simulink model "sysgen_oversample2x_2samples_per_clock"  (R2016b)
settings: Solver=VariableStepAuto  StartTime=0.0  StopTime=samples_per_channel*number_channels/Fadc  RelTol=1e-3
PreLoadFcn:
  | setup
values from neighbouring files (symbols this model uses):
  Fadc = 614e6    (= 614000000)    [setup.m]
undefined symbols (not defined in the file or in its folder): j
libraries: xbsIndex_r4 x434, dspsigops x2, hdlsllib x2
(part 1 of 4)
settings Model: Creator=mdewart  LastModifiedBy=mdewart

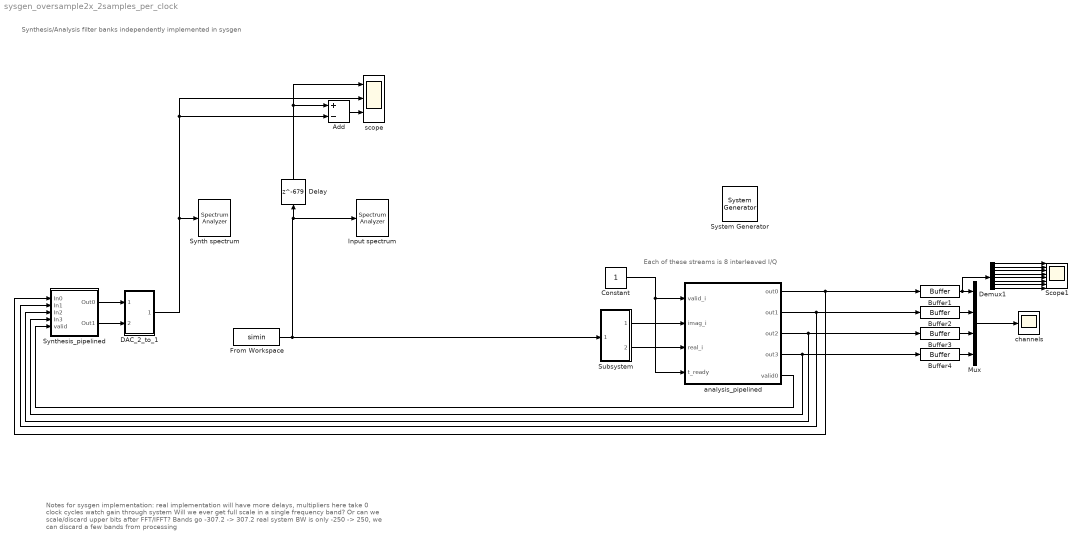
== system sysgen_oversample2x_2samples_per_clock ==
  note: Synthesis/Analysis filter banks independently implemented in sysgen
  note: Notes for sysgen implementation:
      |
      | real implementation will have more delays, multipliers here take 0 clock cycles
      |
      | watch gain through system
      |      Will we ever get full scale in a single frequency band?  Or can we scale/discard upper bits after FFT/IFFT?
      |
      | Bands go -307.2 -> 307.2  real system BW is only -250 -> 250, we can discard a few bands from processing
  note: Each of these streams is 8 interleaved I/Q
  " System Generator" : xbsIndex_r4/ System Generator  Tag=genX  xilinxfamily=kintexu  part=xcku040  speed=-2-e  package=ffva1156  synthesis_tool=Vivado  clock_wrapper=Clock Enables  directory=./netlist  proj_type=Vivado  Synth_file=Vivado Synthesis Defaults  Impl_file=Vivado Implementation Defaults  testbench=off  simulink_period=2/Fadc  sysclk_period=2e9/Fadc  dcm_input_clock_period=10  incr_netlist=off  trim_vbits=Everywhere in SubSystem  dbl_ovrd=According to Block Masks  core_generation=According to Block Masks  run_coregen=off  deprecated_control=off  eval_field=0  block_type=sysgen
  Add : Sum  Inputs=+-
  Buffer{1..4} (4 alike) : Buffer  N=8  TreatMby1Signals=One channel  OutputFrames=off
  Constant : Constant  SampleTime=2/Fadc
  DAC_2_to_1 : Subsystem
  Delay : Delay  DelayLength=679  InitialCondition=0
  Demux1 : Demux  Outputs=8
  From Workspace : FromWorkspace  VariableName=simin  SampleTime=1/Fadc  Interpolate=off  OutputAfterFinalValue=Cyclic repetition
  Input spectrum : SpectrumAnalyzer
  Mux : Mux
  Scope1 : Scope  NumInputPorts=8
  Subsystem : Subsystem
  Synth spectrum : SpectrumAnalyzer
  Synthesis_pipelined : Subsystem  VariantControl=Variant
  analysis_pipelined : Subsystem
  channels : Scope
  scope : Scope  NumInputPorts=3
  wires:
  Mux/1 -> channels/1
  Buffer2/1 -> Mux/2
  Buffer3/1 -> Mux/3
  Buffer4/1 -> Mux/4
  DAC_2_to_1/1(Out1) -> scope/2, Add/2, Synth spectrum/1
  Delay/1 -> Add/1, scope/1
  Subsystem/1(imag) -> analysis_pipelined/2(imag_i)
  Subsystem/2(real) -> analysis_pipelined/3(real_i)
  Constant/1 -> analysis_pipelined/4(t_ready), analysis_pipelined/1(valid_i)
  Buffer1/1 -> Demux1/1, Mux/1
  From Workspace/1 -> Input spectrum/1, Delay/1, Subsystem/1(In1)
  Demux1/1 -> Scope1/1
  Demux1/2 -> Scope1/2
  Demux1/3 -> Scope1/3
  Demux1/4 -> Scope1/4
  Demux1/5 -> Scope1/5
  Demux1/6 -> Scope1/6
  Demux1/7 -> Scope1/7
  Demux1/8 -> Scope1/8
  analysis_pipelined/3(out2) -> Synthesis_pipelined/3(In2), Buffer3/1
  analysis_pipelined/4(out3) -> Synthesis_pipelined/4(In3), Buffer4/1
  analysis_pipelined/2(out1) -> Synthesis_pipelined/2(In1), Buffer2/1
  analysis_pipelined/1(out0) -> Synthesis_pipelined/1(In0), Buffer1/1
  Synthesis_pipelined/1(Out0) -> DAC_2_to_1/1(In1)
  Synthesis_pipelined/2(Out1) -> DAC_2_to_1/2(In2)
  analysis_pipelined/5(valid0) -> Synthesis_pipelined/5(valid)
  Add/1 -> scope/3

== system sysgen_oversample2x_2samples_per_clock/DAC_2_to_1 ==
  In1 : Inport
  In2 : Inport  Port=2
  Add2 : Sum
  Delay7 : Delay  DelayLength=1  InitialCondition=0
  Gain : Gain  Gain=16
  Upsample1 : dspsigops/Upsample  N=2  phase=0  RateOptions=Allow multirate processing  ic=0  mode=Unused parameter value
  Upsample2 : dspsigops/Upsample  N=2  phase=0  RateOptions=Allow multirate processing  ic=0  mode=Unused parameter value
  Out1 : Outport
  wires:
  In2/1 -> Upsample2/1
  Delay7/1 -> Add2/2
  In1/1 -> Upsample1/1
  Upsample1/1 -> Add2/1
  Add2/1 -> Gain/1
  Upsample2/1 -> Delay7/1
  Gain/1 -> Out1/1

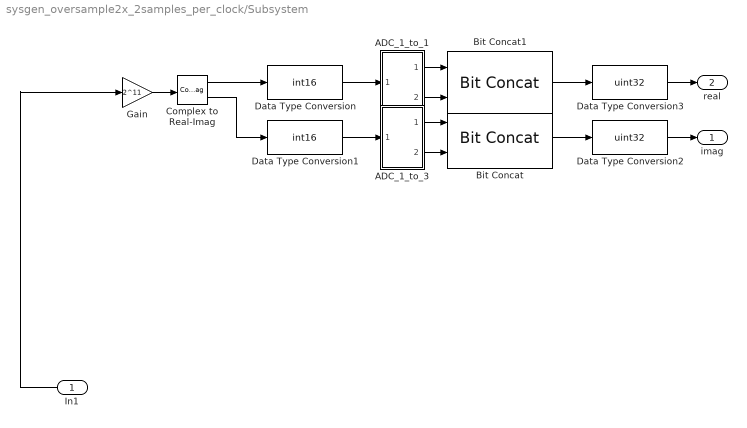
== system sysgen_oversample2x_2samples_per_clock/Subsystem ==
  In1 : Inport
  ADC_1_to_1 : Subsystem
  ADC_1_to_3 : Subsystem
  Bit Concat : hdlsllib/HDL Operations/Bit Concat  numInputs=2
  Bit Concat1 : hdlsllib/HDL Operations/Bit Concat  numInputs=2
  Complex to Real-Imag : ComplexToRealImag
  Data Type Conversion : DataTypeConversion  OutDataTypeStr=int16
  Data Type Conversion1 : DataTypeConversion  OutDataTypeStr=int16
  Data Type Conversion2 : DataTypeConversion  OutDataTypeStr=uint32  ConvertRealWorld=Stored Integer (SI)
  Data Type Conversion3 : DataTypeConversion  OutDataTypeStr=uint32  ConvertRealWorld=Stored Integer (SI)
  Gain : Gain  Gain=2^11
  imag : Outport
  real : Outport  Port=2
  wires:
  In1/1 -> Gain/1
  Data Type Conversion/1 -> ADC_1_to_1/1(In1)
  Complex to Real-Imag/1 -> Data Type Conversion/1
  ADC_1_to_3/2(Out2) -> Bit Concat/2
  Data Type Conversion1/1 -> ADC_1_to_3/1(In1)
  ADC_1_to_1/1(Out1) -> Bit Concat1/1
  Bit Concat/1 -> Data Type Conversion2/1
  ADC_1_to_3/1(Out1) -> Bit Concat/1
  ADC_1_to_1/2(Out2) -> Bit Concat1/2
  Complex to Real-Imag/2 -> Data Type Conversion1/1
  Gain/1 -> Complex to Real-Imag/1
  Bit Concat1/1 -> Data Type Conversion3/1
  Data Type Conversion2/1 -> imag/1
  Data Type Conversion3/1 -> real/1

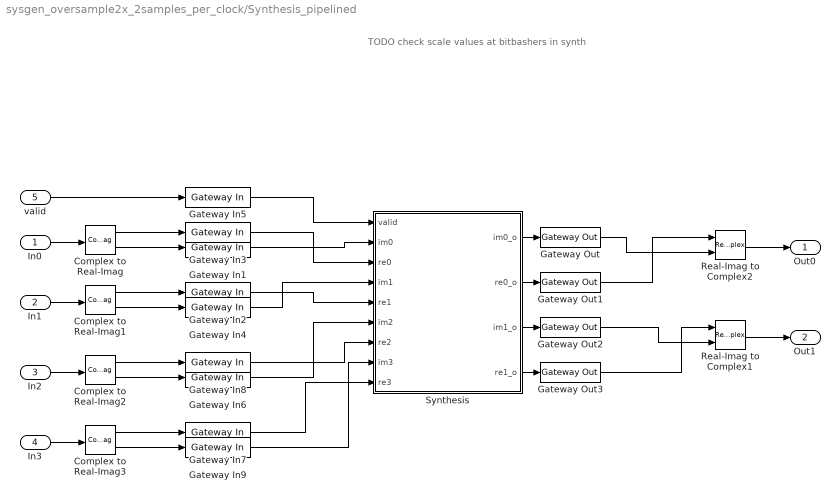
== system sysgen_oversample2x_2samples_per_clock/Synthesis_pipelined ==
  note: TODO check scale values at bitbashers in synth
  In0 : Inport
  In1 : Inport  Port=2
  In2 : Inport  Port=3
  In3 : Inport  Port=4
  valid : Inport  Port=5
  Complex to Real-Imag{,1..3} (4 alike) : ComplexToRealImag
  Gateway In{1..4,6..9} (8 alike) : xbsIndex_r4/Gateway In  gui_display_data_type=Fixed-point  arith_type="Signed  (2's comp)"  n_bits=16  bin_pt=15  preci_type=Single  exp_width=8  frac_width=24  rows=1  columns=1  quantization="Round  (unbiased: +/- Inf)"  overflow=Saturate  period=2/Fadc  UseAsADC=off  ADCChannel='1'  interface=None  automatic_assignment=on  address_offset=hex2dec('00')  intf_name=''  intf_description=''  default_value=0  timing_constraint=None  locs_specified=off  LOCs={}  io_standard={}  inherit_from_input=off  hdl_port=on  dbl_ovrd=off  block_type=gatewayin
  Gateway In5 : xbsIndex_r4/Gateway In  gui_display_data_type=Boolean  arith_type=Boolean  n_bits=1  bin_pt=0  preci_type=Single  exp_width=8  frac_width=24  rows=1  columns=1  quantization="Round  (unbiased: +/- Inf)"  overflow=Saturate  period=2/Fadc  UseAsADC=off  ADCChannel='1'  interface=None  automatic_assignment=on  address_offset=hex2dec('00')  intf_name=''  intf_description=''  default_value=0  timing_constraint=None  locs_specified=off  LOCs={}  io_standard={}  inherit_from_input=off  hdl_port=on  dbl_ovrd=off  block_type=gatewayin
  Gateway Out{,1..3} (4 alike) : xbsIndex_r4/Gateway Out  inherit_from_input=off  hdl_port=on  rows=1  columns=1  UseAsDAC=off  DACChannel='1'  interface=None  automatic_assignment=on  address_offset=hex2dec('00')  intf_name=''  intf_description=''  timing_constraint=None  locs_specified=off  LOCs={}  io_standard={}  block_type=gatewayout
  Real-Imag to Complex1 : RealImagToComplex
  Real-Imag to Complex2 : RealImagToComplex
  Synthesis : Subsystem
  Out0 : Outport
  Out1 : Outport  Port=2
  wires:
  Real-Imag to Complex1/1 -> Out1/1
  Real-Imag to Complex2/1 -> Out0/1
  Gateway Out3/1 -> Real-Imag to Complex1/1
  Gateway Out2/1 -> Real-Imag to Complex1/2
  Gateway Out/1 -> Real-Imag to Complex2/2
  Gateway Out1/1 -> Real-Imag to Complex2/1
  Synthesis/4(re1_o) -> Gateway Out3/1
  Synthesis/3(im1_o) -> Gateway Out2/1
  Synthesis/2(re0_o) -> Gateway Out1/1
  Synthesis/1(im0_o) -> Gateway Out/1
  Gateway In7/1 -> Synthesis/9(re3)
  Gateway In9/1 -> Synthesis/8(im3)
  Gateway In8/1 -> Synthesis/7(re2)
  Gateway In6/1 -> Synthesis/6(im2)
  Gateway In4/1 -> Synthesis/4(im1)
  Gateway In2/1 -> Synthesis/5(re1)
  Gateway In5/1 -> Synthesis/1(valid)
  Gateway In1/1 -> Synthesis/2(im0)
  Gateway In3/1 -> Synthesis/3(re0)
  In2/1 -> Complex to Real-Imag2/1
  In3/1 -> Complex to Real-Imag3/1
  Complex to Real-Imag3/2 -> Gateway In9/1
  Complex to Real-Imag3/1 -> Gateway In7/1
  Complex to Real-Imag2/2 -> Gateway In6/1
  Complex to Real-Imag2/1 -> Gateway In8/1
  In0/1 -> Complex to Real-Imag/1
  In1/1 -> Complex to Real-Imag1/1
  Complex to Real-Imag1/2 -> Gateway In4/1
  Complex to Real-Imag1/1 -> Gateway In2/1
  Complex to Real-Imag/2 -> Gateway In1/1
  Complex to Real-Imag/1 -> Gateway In3/1
  valid/1 -> Gateway In5/1

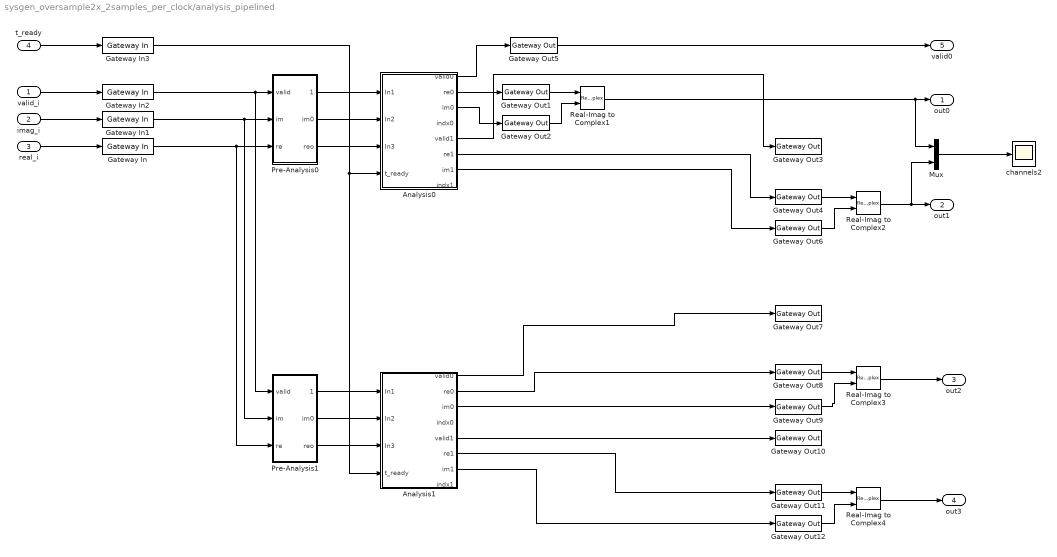
== system sysgen_oversample2x_2samples_per_clock/analysis_pipelined ==
  valid_i : Inport
  imag_i : Inport  Port=2
  real_i : Inport  Port=3
  t_ready : Inport  Port=4
  Analysis0 : Subsystem
  Analysis1 : Subsystem
  Gateway In : xbsIndex_r4/Gateway In  gui_display_data_type=Fixed-point  arith_type=Unsigned  n_bits=32  bin_pt=0  preci_type=Single  exp_width=8  frac_width=24  rows=1  columns=1  quantization="Round  (unbiased: +/- Inf)"  overflow=Saturate  period=2/Fadc  UseAsADC=off  ADCChannel='1'  interface=None  automatic_assignment=on  address_offset=hex2dec('00')  intf_name=''  intf_description=''  default_value=0  timing_constraint=None  locs_specified=off  LOCs={}  io_standard={}  inherit_from_input=off  hdl_port=on  dbl_ovrd=off  block_type=gatewayin
  Gateway In1 : xbsIndex_r4/Gateway In  gui_display_data_type=Fixed-point  arith_type=Unsigned  n_bits=32  bin_pt=0  preci_type=Single  exp_width=8  frac_width=24  rows=1  columns=1  quantization="Round  (unbiased: +/- Inf)"  overflow=Saturate  period=2/Fadc  UseAsADC=off  ADCChannel='1'  interface=None  automatic_assignment=on  address_offset=hex2dec('00')  intf_name=''  intf_description=''  default_value=0  timing_constraint=None  locs_specified=off  LOCs={}  io_standard={}  inherit_from_input=off  hdl_port=on  dbl_ovrd=off  block_type=gatewayin
  Gateway In2 : xbsIndex_r4/Gateway In  gui_display_data_type=Boolean  arith_type=Boolean  n_bits=1  bin_pt=0  preci_type=Single  exp_width=8  frac_width=24  rows=1  columns=1  quantization="Round  (unbiased: +/- Inf)"  overflow=Saturate  period=2/Fadc  UseAsADC=off  ADCChannel='1'  interface=None  automatic_assignment=on  address_offset=hex2dec('00')  intf_name=''  intf_description=''  default_value=0  timing_constraint=None  locs_specified=off  LOCs={}  io_standard={}  inherit_from_input=off  hdl_port=on  dbl_ovrd=off  block_type=gatewayin
  Gateway In3 : xbsIndex_r4/Gateway In  gui_display_data_type=Boolean  arith_type=Boolean  n_bits=1  bin_pt=0  preci_type=Single  exp_width=8  frac_width=24  rows=1  columns=1  quantization="Round  (unbiased: +/- Inf)"  overflow=Saturate  period=2/Fadc  UseAsADC=off  ADCChannel='1'  interface=None  automatic_assignment=on  address_offset=hex2dec('00')  intf_name=''  intf_description=''  default_value=0  timing_constraint=None  locs_specified=off  LOCs={}  io_standard={}  inherit_from_input=off  hdl_port=on  dbl_ovrd=off  block_type=gatewayin
  Gateway Out{1..12} (12 alike) : xbsIndex_r4/Gateway Out  inherit_from_input=off  hdl_port=on  rows=1  columns=1  UseAsDAC=off  DACChannel='1'  interface=None  automatic_assignment=on  address_offset=hex2dec('00')  intf_name=''  intf_description=''  timing_constraint=None  locs_specified=off  LOCs={}  io_standard={}  block_type=gatewayout
  Mux : Mux  Inputs=2
  Pre-Analysis0 : Subsystem
  Pre-Analysis1 : Subsystem
  Real-Imag to Complex{1..4} (4 alike) : RealImagToComplex
  channels2 : Scope
  out0 : Outport
  out1 : Outport  Port=2
  out2 : Outport  Port=3
  out3 : Outport  Port=4
  valid0 : Outport  Port=5
  wires:
  Gateway In2/1 -> Pre-Analysis0/1(valid), Pre-Analysis1/1(valid)
  Analysis1/7(im1) -> Gateway Out12/1
  Analysis1/6(re1) -> Gateway Out11/1
  Analysis1/3(im0) -> Gateway Out9/1
  Analysis0/1(valid0) -> Gateway Out5/1
  Analysis0/2(re0) -> Gateway Out1/1
  Analysis0/3(im0) -> Gateway Out2/1
  Real-Imag to Complex4/1 -> out3/1
  Real-Imag to Complex3/1 -> out2/1
  Real-Imag to Complex1/1 -> Mux/1, out0/1
  Gateway Out5/1 -> valid0/1
  Pre-Analysis1/1(valid0) -> Analysis1/1(In1)
  Pre-Analysis1/2(im0) -> Analysis1/2(In2)
  Pre-Analysis1/3(reo) -> Analysis1/3(In3)
  Gateway In3/1 -> Analysis0/4(t_ready), Analysis1/4(t_ready)
  Pre-Analysis0/1(valid0) -> Analysis0/1(In1)
  Pre-Analysis0/2(im0) -> Analysis0/2(In2)
  Pre-Analysis0/3(reo) -> Analysis0/3(In3)
  Gateway In/1 -> Pre-Analysis0/3(re), Pre-Analysis1/3(re)
  Gateway In1/1 -> Pre-Analysis0/2(im), Pre-Analysis1/2(im)
  Analysis1/5(valid1) -> Gateway Out10/1
  Analysis1/2(re0) -> Gateway Out8/1
  Analysis1/1(valid0) -> Gateway Out7/1
  Gateway Out9/1 -> Real-Imag to Complex3/2
  Gateway Out8/1 -> Real-Imag to Complex3/1
  Gateway Out12/1 -> Real-Imag to Complex4/2
  Gateway Out11/1 -> Real-Imag to Complex4/1
  Analysis0/7(im1) -> Gateway Out6/1
  Analysis0/6(re1) -> Gateway Out4/1
  Analysis0/5(valid1) -> Gateway Out3/1
  Gateway Out2/1 -> Real-Imag to Complex1/2
  Gateway Out1/1 -> Real-Imag to Complex1/1
  Gateway Out6/1 -> Real-Imag to Complex2/2
  Gateway Out4/1 -> Real-Imag to Complex2/1
  imag_i/1 -> Gateway In1/1
  real_i/1 -> Gateway In/1
  t_ready/1 -> Gateway In3/1
  valid_i/1 -> Gateway In2/1
  Real-Imag to Complex2/1 -> Mux/2, out1/1
  Mux/1 -> channels2/1

== system sysgen_oversample2x_2samples_per_clock/Subsystem/ADC_1_to_1 ==
  In1 : Inport
  Delay1 : Delay  DelayLength=1  InitialCondition=0
  Downsample : DownSample  RateOptions=Allow multirate processing
  Downsample1 : DownSample  RateOptions=Allow multirate processing
  Out1 : Outport
  Out2 : Outport  Port=2
  wires:
  Downsample/1 -> Out2/1
  In1/1 -> Downsample/1, Delay1/1
  Downsample1/1 -> Out1/1
  Delay1/1 -> Downsample1/1

== system sysgen_oversample2x_2samples_per_clock/Subsystem/ADC_1_to_3 ==
  In1 : Inport
  Delay1 : Delay  DelayLength=1  InitialCondition=0
  Downsample : DownSample  RateOptions=Allow multirate processing
  Downsample1 : DownSample  RateOptions=Allow multirate processing
  Out1 : Outport
  Out2 : Outport  Port=2
  wires:
  Delay1/1 -> Downsample1/1
  Downsample1/1 -> Out1/1
  In1/1 -> Delay1/1, Downsample/1
  Downsample/1 -> Out2/1

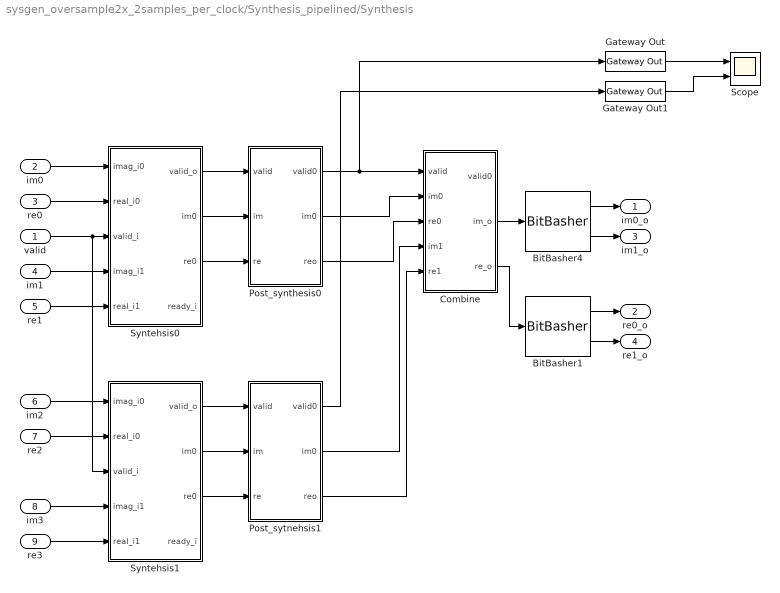
== system sysgen_oversample2x_2samples_per_clock/Synthesis_pipelined/Synthesis ==
  valid : Inport
  im0 : Inport  Port=2
  re0 : Inport  Port=3
  im1 : Inport  Port=4
  re1 : Inport  Port=5
  im2 : Inport  Port=6
  re2 : Inport  Port=7
  im3 : Inport  Port=8
  re3 : Inport  Port=9
  BitBasher1 : xbsIndex_r4/BitBasher  bitexpr=|  display_expr=off  sr_1=hi  arith_type1="Signed  (2's comp)"  bin_pt1=15  sr_2=lo  arith_type2="Signed  (2's comp)"  bin_pt2=15  sr_3=hi  arith_type3=Unsigned  bin_pt3=0  sr_4=4  arith_type4=Unsigned  bin_pt4=0  dbl_ovrd=off  block_type=bitbasher
      | hi = {in[31:16]}
      | lo = {in[15:0]}
  BitBasher4 : xbsIndex_r4/BitBasher  bitexpr=|  display_expr=off  sr_1=hi  arith_type1="Signed  (2's comp)"  bin_pt1=15  sr_2=lo  arith_type2="Signed  (2's comp)"  bin_pt2=15  sr_3=hi  arith_type3=Unsigned  bin_pt3=0  sr_4=4  arith_type4=Unsigned  bin_pt4=0  dbl_ovrd=off  block_type=bitbasher
      | hi = {in[31:16]}
      | lo = {in[15:0]}
  Combine : Subsystem
  Gateway Out : xbsIndex_r4/Gateway Out  inherit_from_input=off  hdl_port=off  rows=1  columns=1  UseAsDAC=off  DACChannel='1'  interface=None  automatic_assignment=on  address_offset=hex2dec('00')  intf_name=''  intf_description=''  timing_constraint=None  locs_specified=off  LOCs={}  io_standard={}  block_type=gatewayout
  Gateway Out1 : xbsIndex_r4/Gateway Out  inherit_from_input=off  hdl_port=off  rows=1  columns=1  UseAsDAC=off  DACChannel='1'  interface=None  automatic_assignment=on  address_offset=hex2dec('00')  intf_name=''  intf_description=''  timing_constraint=None  locs_specified=off  LOCs={}  io_standard={}  block_type=gatewayout
  Post_synthesis0 : Subsystem
  Post_sytnehsis1 : Subsystem
  Scope : Scope  NumInputPorts=2
  Syntehsis0 : Subsystem
  Syntehsis1 : Subsystem
  im0_o : Outport
  re0_o : Outport  Port=2
  im1_o : Outport  Port=3
  re1_o : Outport  Port=4
  wires:
  Post_sytnehsis1/1(valid0) -> Gateway Out1/1
  Gateway Out1/1 -> Scope/2
  Gateway Out/1 -> Scope/1
  Syntehsis0/1(valid_o) -> Post_synthesis0/1(valid)
  BitBasher1/2 -> re1_o/1
  BitBasher1/1 -> re0_o/1
  BitBasher4/2 -> im1_o/1
  BitBasher4/1 -> im0_o/1
  Combine/3(re_o) -> BitBasher1/1
  Combine/2(im_o) -> BitBasher4/1
  Post_sytnehsis1/3(reo) -> Combine/5(re1)
  Post_sytnehsis1/2(im0) -> Combine/4(im1)
  Post_synthesis0/3(reo) -> Combine/3(re0)
  Post_synthesis0/2(im0) -> Combine/2(im0)
  Post_synthesis0/1(valid0) -> Combine/1(valid), Gateway Out/1
  Syntehsis0/3(re0) -> Post_synthesis0/3(re)
  Syntehsis0/2(im0) -> Post_synthesis0/2(im)
  Syntehsis1/1(valid_o) -> Post_sytnehsis1/1(valid)
  Syntehsis1/3(re0) -> Post_sytnehsis1/3(re)
  Syntehsis1/2(im0) -> Post_sytnehsis1/2(im)
  im3/1 -> Syntehsis1/4(imag_i1)
  re1/1 -> Syntehsis0/5(real_i1)
  valid/1 -> Syntehsis1/3(valid_i), Syntehsis0/3(valid_i)
  re3/1 -> Syntehsis1/5(real_i1)
  im1/1 -> Syntehsis0/4(imag_i1)
  im0/1 -> Syntehsis0/1(imag_i0)
  re0/1 -> Syntehsis0/2(real_i0)
  re2/1 -> Syntehsis1/2(real_i0)
  im2/1 -> Syntehsis1/1(imag_i0)

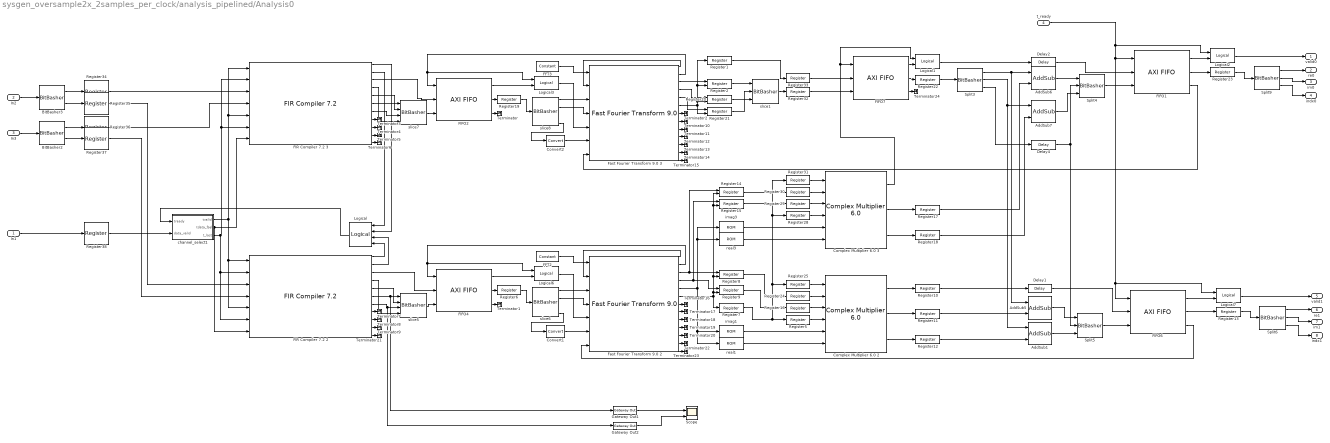
== system sysgen_oversample2x_2samples_per_clock/analysis_pipelined/Analysis0 ==
  In1 : Inport
  In2 : Inport  Port=2
  In3 : Inport  Port=3
  t_ready : Inport  Port=4
  AddSub{1,5..7} (4 alike) : xbsIndex_r4/AddSub  mode=Addition  use_carryin=off  use_carryout=off  en=off  latency=2  precision=Full  arith_type="Signed  (2's comp)"  n_bits=22  bin_pt=16  quantization=Truncate  overflow=Wrap  use_behavioral_HDL=on  hw_selection=Fabric  pipelined=off  dbl_ovrd=off  block_type=addsub
  BitBasher2 : xbsIndex_r4/BitBasher  bitexpr=|  display_expr=off  sr_1=hi  arith_type1="Signed  (2's comp)"  bin_pt1=15  sr_2=lo  arith_type2="Signed  (2's comp)"  bin_pt2=15  sr_3=hi  arith_type3=Unsigned  bin_pt3=0  sr_4=4  arith_type4=Unsigned  bin_pt4=0  dbl_ovrd=off  block_type=bitbasher
      | hi = {in[31:16]}
      | lo = {in[15:0]}
  BitBasher3 : xbsIndex_r4/BitBasher  bitexpr=|  display_expr=off  sr_1=hi  arith_type1="Signed  (2's comp)"  bin_pt1=15  sr_2=lo  arith_type2="Signed  (2's comp)"  bin_pt2=15  sr_3=hi  arith_type3=Unsigned  bin_pt3=0  sr_4=4  arith_type4=Unsigned  bin_pt4=0  dbl_ovrd=off  block_type=bitbasher
      | hi = {in[31:16]}
      | lo = {in[15:0]}
  Complex Multiplier 6.0 2 : xbsIndex_r4/Complex Multiplier 6.0   hasatlast=off  hasatuser=off  atuserwidth=1  hasbtlast=off  hasbtuser=off  btuserwidth=1  multtype=Use_Mults  optimizegoal=Performance  flowcontrol=NonBlocking  outputwidth=24  roundmode=Truncate  hasctrltlast=off  hasctrltuser=off  ctrltuserwidth=1  outtlastbehv=Null  latencyconfig=Automatic  minimumlatency=34  aclken=off  aresetn=off  trim_axipin_name=on  simulation_type=hybrid_sim  simulation_model=sysgen:cmpy_v6_0  data_path_portlist={ 's_axis_a_tdata_real', 's_axis_a_tdata_imag', 's_axis_b_tdata_real', 's_axis_b_tdata_imag', 's_axis_ctrl_tdata_rounding_bit', 'm_axis_dout_tdata_real', 'm_axis_dout_tdata_imag' }  aportwidth=63  bportwidth=63  ip_name=Complex Multiplier  ip_version=6.0  dsptool_ready=true  ipcore_usecache=true  ipcore_useipmodelcache=true  ipcore_verbose=false  ipcore_latency_parameter='minimumlatency'  wrapper_available=true  port_translation_map={ 'aclken' => 'en', 'aresetn' => 'rst'}  block_type=cmpy_v6_0
  Complex Multiplier 6.0 3 : xbsIndex_r4/Complex Multiplier 6.0   hasatlast=off  hasatuser=off  atuserwidth=1  hasbtlast=off  hasbtuser=off  btuserwidth=1  multtype=Use_Mults  optimizegoal=Performance  flowcontrol=NonBlocking  outputwidth=24  roundmode=Truncate  hasctrltlast=off  hasctrltuser=off  ctrltuserwidth=1  outtlastbehv=Null  latencyconfig=Automatic  minimumlatency=34  aclken=off  aresetn=off  trim_axipin_name=on  simulation_type=hybrid_sim  simulation_model=sysgen:cmpy_v6_0  data_path_portlist={ 's_axis_a_tdata_real', 's_axis_a_tdata_imag', 's_axis_b_tdata_real', 's_axis_b_tdata_imag', 's_axis_ctrl_tdata_rounding_bit', 'm_axis_dout_tdata_real', 'm_axis_dout_tdata_imag' }  aportwidth=63  bportwidth=63  ip_name=Complex Multiplier  ip_version=6.0  dsptool_ready=true  ipcore_usecache=true  ipcore_useipmodelcache=true  ipcore_verbose=false  ipcore_latency_parameter='minimumlatency'  wrapper_available=true  port_translation_map={ 'aclken' => 'en', 'aresetn' => 'rst'}  block_type=cmpy_v6_0
  Convert1 : xbsIndex_r4/Convert  gui_display_data_type=Boolean  arith_type=Boolean  n_bits=16  bin_pt=15  float_type=Single  exp_bits=8  fraction_bits=24  quantization=Truncate  overflow=Flag as error  en=off  latency=0  pipeline=off  dbl_ovrd=off  block_type=convert
  Convert2 : xbsIndex_r4/Convert  gui_display_data_type=Boolean  arith_type=Boolean  n_bits=16  bin_pt=15  float_type=Single  exp_bits=8  fraction_bits=24  quantization=Truncate  overflow=Flag as error  en=off  latency=0  pipeline=off  dbl_ovrd=off  block_type=convert
  Delay1 : xbsIndex_r4/Delay  rst=off  infoeditControl=Selection of Reset will increase slice count due to use of real FFs and instead of SRLs  en=off  latency=2  reg_retiming=on  dbl_ovrd=off  block_type=delay
  Delay2 : xbsIndex_r4/Delay  rst=off  infoeditControl=Selection of Reset will increase slice count due to use of real FFs and instead of SRLs  en=off  latency=2  reg_retiming=on  dbl_ovrd=off  block_type=delay
  Delay4 : xbsIndex_r4/Delay  rst=off  infoeditControl=Selection of Reset will increase slice count due to use of real FFs and instead of SRLs  en=off  latency=2  reg_retiming=on  dbl_ovrd=off  block_type=delay
  FFT2 : xbsIndex_r4/Constant  const=1  gui_display_data_type=Fixed-point  arith_type=Unsigned  n_bits=1  bin_pt=0  preci_type=Single  exp_width=8  frac_width=24  explicit_period=off  period=1  equ=P=C  opselect=C  inp2=PCIN>>17  opr=+  inp1=P  carry=CIN  dbl_ovrd=off  block_type=constant
  FFT3 : xbsIndex_r4/Constant  const=1  gui_display_data_type=Fixed-point  arith_type=Unsigned  n_bits=1  bin_pt=0  preci_type=Single  exp_width=8  frac_width=24  explicit_period=off  period=1  equ=P=C  opselect=C  inp2=PCIN>>17  opr=+  inp1=P  carry=CIN  dbl_ovrd=off  block_type=constant
  FIFO{1..2,4,6} (4 alike) : xbsIndex_r4/AXI FIFO  input_depth_axis=16  actual_fifo_depth_label=18  enable_tdata=on  enable_tdest=off  enable_tstrb=off  enable_tready=on  enable_tid=off  enable_tuser=off  enable_tkeep=off  enable_tlast=off  has_aresetn=off  enable_data_counts_axis=off  fifo_implementation_type_axis=Common Clock Distributed RAM  trim_axipin_name=on  programmable_full_type_axis=Full  full_threshold_assert_value_axis=0  programmable_empty_type_axis=Empty  empty_threshold_assert_value_axis=1022  underflow_flag_axi=0  underflow_sense_axi=Active High  overflow_flag_axi=0  overflow_sense_axi=Active High  block_type=axi_fifo
  FIFO7 : xbsIndex_r4/AXI FIFO  input_depth_axis=32  actual_fifo_depth_label=34  enable_tdata=on  enable_tdest=off  enable_tstrb=off  enable_tready=on  enable_tid=off  enable_tuser=off  enable_tkeep=off  enable_tlast=off  has_aresetn=off  enable_data_counts_axis=off  fifo_implementation_type_axis=Common Clock Distributed RAM  trim_axipin_name=on  programmable_full_type_axis=Full  full_threshold_assert_value_axis=0  programmable_empty_type_axis=Empty  empty_threshold_assert_value_axis=1022  underflow_flag_axi=0  underflow_sense_axi=Active High  overflow_flag_axi=0  overflow_sense_axi=Active High  block_type=axi_fifo
  FIR Compiler 7.2 2 : xbsIndex_r4/FIR Compiler 7.2   coefficientvector=analysis_coefficients2  coefficient_sets=8  coefficient_reload=off  filter_type=Single_Rate  rate_change_type=Integer  interpolation_rate=1  decimation_rate=1  zero_pack_factor=1  channel_sequence=Basic  number_channels=8  pattern_list='P4-0,P4-1,P4-2,P4-3,P4-4'  number_paths=2  ratespecification=Output_Sample_Period  sampleperiod=1.00000000  hardwareoversamplingrate=1  coefficient_sign=Signed  quantization=Quantize_Only  coefficient_width=25  bestprecision=on  coefficient_fractional_bits=28  coefficient_structure=Inferred  output_rounding_mode=Convergent_Rounding_to_Even  output_width=19  filter_architecture=Systolic_Multiply_Accumulate  optimization_goal=Area  optimization_list='None'  data_buffer_type=Automatic  coefficient_buffer_type=Automatic  input_buffer_type=Automatic  output_buffer_type=Automatic  preference_for_other_storage=Automatic  multi_column_support=Automatic  columnconfig='16'  inter_column_pipe_length=4  data_has_tlast=Vector_Framing  m_data_has_tready=off  s_data_has_fifo=off  s_data_has_tuser=Not_Required  m_data_has_tuser=Chan_ID_Field  s_config_sync_mode=On_Vector  s_config_method=By_Channel  num_reload_slots=1  has_aclken=off  has_aresetn=off  infoeditControl=ARESETn must be asserted for a minimum of 2 cycles  reset_data_vector=on  trim_axipin_name=on  simulation_type=hybrid_sim  simulation_model=sysgen:xfirv7_2_cmodel  data_path_portlist={ 's_axis_data_tdata', 'm_axis_data_tdata' }  passband_min=0.0  passband_max=0.5  stopband_min=0.5  stopband_max=1.0  filter_selection=1  gui_behaviour='Sysgen_GUI'  data_sign=Signed  data_width=16  data_fractional_bits=0  data_tuser_width=1  wrapper_available=true  ip_wrap_arbitrary_binary_point=true  ip_name=FIR Compiler  ip_version=7.2  dsptool_ready=true  ipcore_usecache=true  ipcore_useipmodelcache=true  port_translation_map={ 'aclken' => 'en', 'aresetn' => 'rst' }  run_core_at_system_period=true  ipcore_xco_need_fpga_part=true  block_type=fir_compiler_v7_2
      settings: infoedit=Maximum Possible : Maximizes oversampling rate. Abstracted input handshake (no s_data_tvalid) and automatic rate propagation.<br>Hardware Oversampling Rate : Specifies oversampling rate relative to the input sample period. Abstracted input handshake (no s_data_tvalid) and automatic rate propagation.<br>Input/Output Sample Period : Specifies absolute oversampling rate. No input handshake abstraction (exposes s_data_tvalid) and no rate propagation.
  FIR Compiler 7.2 3 : xbsIndex_r4/FIR Compiler 7.2   coefficientvector=analysis_coefficients1  coefficient_sets=8  coefficient_reload=off  filter_type=Single_Rate  rate_change_type=Integer  interpolation_rate=1  decimation_rate=1  zero_pack_factor=1  channel_sequence=Basic  number_channels=8  pattern_list='P4-0,P4-1,P4-2,P4-3,P4-4'  number_paths=2  ratespecification=Output_Sample_Period  sampleperiod=1.00000000  hardwareoversamplingrate=1  coefficient_sign=Signed  quantization=Quantize_Only  coefficient_width=25  bestprecision=on  coefficient_fractional_bits=28  coefficient_structure=Inferred  output_rounding_mode=Convergent_Rounding_to_Even  output_width=19  filter_architecture=Systolic_Multiply_Accumulate  optimization_goal=Area  optimization_list='None'  data_buffer_type=Automatic  coefficient_buffer_type=Automatic  input_buffer_type=Automatic  output_buffer_type=Automatic  preference_for_other_storage=Automatic  multi_column_support=Automatic  columnconfig='16'  inter_column_pipe_length=4  data_has_tlast=Vector_Framing  m_data_has_tready=off  s_data_has_fifo=off  s_data_has_tuser=Not_Required  m_data_has_tuser=Chan_ID_Field  s_config_sync_mode=On_Vector  s_config_method=By_Channel  num_reload_slots=1  has_aclken=off  has_aresetn=off  infoeditControl=ARESETn must be asserted for a minimum of 2 cycles  reset_data_vector=on  trim_axipin_name=on  simulation_type=hybrid_sim  simulation_model=sysgen:xfirv7_2_cmodel  data_path_portlist={ 's_axis_data_tdata', 'm_axis_data_tdata' }  passband_min=0.0  passband_max=0.5  stopband_min=0.5  stopband_max=1.0  filter_selection=1  gui_behaviour='Sysgen_GUI'  data_sign=Signed  data_width=16  data_fractional_bits=0  data_tuser_width=1  wrapper_available=true  ip_wrap_arbitrary_binary_point=true  ip_name=FIR Compiler  ip_version=7.2  dsptool_ready=true  ipcore_usecache=true  ipcore_useipmodelcache=true  port_translation_map={ 'aclken' => 'en', 'aresetn' => 'rst' }  run_core_at_system_period=true  ipcore_xco_need_fpga_part=true  block_type=fir_compiler_v7_2
      settings: infoedit=Maximum Possible : Maximizes oversampling rate. Abstracted input handshake (no s_data_tvalid) and automatic rate propagation.<br>Hardware Oversampling Rate : Specifies oversampling rate relative to the input sample period. Abstracted input handshake (no s_data_tvalid) and automatic rate propagation.<br>Input/Output Sample Period : Specifies absolute oversampling rate. No input handshake abstraction (exposes s_data_tvalid) and no rate propagation.
  Fast Fourier Transform 9.0 2 : xbsIndex_r4/Fast Fourier Transform 9.0   transform_length=8  target_clock_frequency=307  target_data_throughput=50  implementation_options=pipelined_streaming_io  run_time_configurable_transform_length=off  phase_factor_width=17  scaling_options=unscaled  rounding_modes=convergent_rounding  aclken=off  aresetn=off  output_ordering=natural_order  cyclic_prefix_insertion=off  throttle_scheme=nonrealtime  xk_index=on  ovflo=off  trim_axipin_name=on  memory_options_data=block_ram  memory_options_phase_factors=block_ram  number_of_stages_using_block_ram_for_data_and_phase_factors=0  memory_options_reorder=block_ram  memory_options_hybrid=off  complex_mult_type=use_mults_performance  butterfly_type=use_xtremedsp_slices  simulation_type=hybrid_sim  simulation_model=sysgen:xfftv9_cmodel  data_path_portlist={ 's_axis_data_tdata', 'm_axis_data_tdata', 'm_axis_status_tdata', 'event_fft_overflow' }  channels=1  input_ordering=natural_order  input_width=16  ip_name=Fast Fourier Transform  ip_version=9.0  dsptool_ready=true  ipcore_usecache=true  ipcore_useipmodelcache=true  wrapper_available=true  port_translation_map={ 'aclken' => 'en', 'aresetn' => 'rst'}  data_format=fixed_point  block_type=xfft_v9_0
  Fast Fourier Transform 9.0 3 : xbsIndex_r4/Fast Fourier Transform 9.0   transform_length=8  target_clock_frequency=307  target_data_throughput=50  implementation_options=pipelined_streaming_io  run_time_configurable_transform_length=off  phase_factor_width=17  scaling_options=unscaled  rounding_modes=convergent_rounding  aclken=off  aresetn=off  output_ordering=natural_order  cyclic_prefix_insertion=off  throttle_scheme=nonrealtime  xk_index=on  ovflo=off  trim_axipin_name=on  memory_options_data=block_ram  memory_options_phase_factors=block_ram  number_of_stages_using_block_ram_for_data_and_phase_factors=0  memory_options_reorder=block_ram  memory_options_hybrid=off  complex_mult_type=use_mults_performance  butterfly_type=use_xtremedsp_slices  simulation_type=hybrid_sim  simulation_model=sysgen:xfftv9_cmodel  data_path_portlist={ 's_axis_data_tdata', 'm_axis_data_tdata', 'm_axis_status_tdata', 'event_fft_overflow' }  channels=1  input_ordering=natural_order  input_width=16  ip_name=Fast Fourier Transform  ip_version=9.0  dsptool_ready=true  ipcore_usecache=true  ipcore_useipmodelcache=true  wrapper_available=true  port_translation_map={ 'aclken' => 'en', 'aresetn' => 'rst'}  data_format=fixed_point  block_type=xfft_v9_0
  Gateway Out1 : xbsIndex_r4/Gateway Out  inherit_from_input=off  hdl_port=off  rows=1  columns=1  UseAsDAC=off  DACChannel='1'  interface=None  automatic_assignment=on  address_offset=hex2dec('00')  intf_name=''  intf_description=''  timing_constraint=None  locs_specified=off  LOCs={}  io_standard={}  block_type=gatewayout
  Gateway Out2 : xbsIndex_r4/Gateway Out  inherit_from_input=off  hdl_port=off  rows=1  columns=1  UseAsDAC=off  DACChannel='1'  interface=None  automatic_assignment=on  address_offset=hex2dec('00')  intf_name=''  intf_description=''  timing_constraint=None  locs_specified=off  LOCs={}  io_standard={}  block_type=gatewayout
  Logical : xbsIndex_r4/Logical  logical_function=AND  inputs=4  en=off  latency=1  precision=Full  arith_type=Unsigned  n_bits=16  bin_pt=0  align_bp=on  dbl_ovrd=off  block_type=logical
  Logical{1..3,6..7} (5 alike) : xbsIndex_r4/Logical  logical_function=AND  inputs=2  en=off  latency=1  precision=Full  arith_type=Unsigned  n_bits=16  bin_pt=0  align_bp=on  dbl_ovrd=off  block_type=logical
  Register{1,5..7,10..13,16..19,22..25,28..38} (27 alike) : xbsIndex_r4/Register  init=0  rst=off  en=off  dbl_ovrd=off  block_type=register
  Register{2,8..9,14..15,20..21} (7 alike) : xbsIndex_r4/Register  init=0  rst=off  en=on  dbl_ovrd=off  block_type=register
  Scope : Scope  NumInputPorts=2
  Split3 : xbsIndex_r4/BitBasher  bitexpr=|  display_expr=off  sr_1=im  arith_type1="Signed  (2's comp)"  bin_pt1=17  sr_2=re  arith_type2="Signed  (2's comp)"  bin_pt2=17  sr_3=indx  arith_type3=Unsigned  bin_pt3=0  sr_4=4  arith_type4=Unsigned  bin_pt4=0  dbl_ovrd=off  block_type=bitbasher
      | im={in[43:22]}
      | re={in[21:0]}
      | indx = {in[46:44]}
  Split4 : xbsIndex_r4/BitBasher  bitexpr=out = {9'b0, indx, im, re}  display_expr=off  sr_1=out  arith_type1="Signed  (2's comp)"  bin_pt1=0  sr_2=im  arith_type2="Signed  (2's comp)"  bin_pt2=18  sr_3=3  arith_type3=Unsigned  bin_pt3=0  sr_4=4  arith_type4=Unsigned  bin_pt4=0  dbl_ovrd=off  block_type=bitbasher
  Split5 : xbsIndex_r4/BitBasher  bitexpr=out = {9'b0, indx, im, re}  display_expr=off  sr_1=out  arith_type1="Signed  (2's comp)"  bin_pt1=0  sr_2=im  arith_type2="Signed  (2's comp)"  bin_pt2=18  sr_3=3  arith_type3=Unsigned  bin_pt3=0  sr_4=4  arith_type4=Unsigned  bin_pt4=0  dbl_ovrd=off  block_type=bitbasher
  Split6 : xbsIndex_r4/BitBasher  bitexpr=|  display_expr=off  sr_1=re  arith_type1="Signed  (2's comp)"  bin_pt1=16  sr_2=im  arith_type2="Signed  (2's comp)"  bin_pt2=16  sr_3=indx  arith_type3=Unsigned  bin_pt3=0  sr_4=4  arith_type4=Unsigned  bin_pt4=0  dbl_ovrd=off  block_type=bitbasher
      | re={in[17:0]}
      | im={in[43:26]}
      | indx ={in[52:54]}
  Split9 : xbsIndex_r4/BitBasher  bitexpr=|  display_expr=off  sr_1=re  arith_type1="Signed  (2's comp)"  bin_pt1=16  sr_2=im  arith_type2="Signed  (2's comp)"  bin_pt2=16  sr_3=indx  arith_type3=Unsigned  bin_pt3=0  sr_4=4  arith_type4=Unsigned  bin_pt4=0  dbl_ovrd=off  block_type=bitbasher
      | re={in[17:0]}
      | im={in[43:26]}
      | indx ={in[54:52]}
  Terminator{,1..24} (25 alike) : Terminator
  channel_select1 : Subsystem
  imag1 : xbsIndex_r4/ROM  depth=8  initVector=imag(exp(-j*2*pi*(8:15)/16))  distributed_mem=Block RAM  rst=off  init_reg=0  en=off  latency=2  gui_display_data_type=Fixed-point  arith_type="Signed  (2's comp)"  n_bits=18  bin_pt=16  preci_type=Single  exp_width=8  frac_width=24  optimize=Area  use_rpm=on  dbl_ovrd=off  block_type=sprom
  imag3 : xbsIndex_r4/ROM  depth=8  initVector=imag(exp(-j*2*pi*(0:7)/16))  distributed_mem=Block RAM  rst=off  init_reg=0  en=off  latency=2  gui_display_data_type=Fixed-point  arith_type="Signed  (2's comp)"  n_bits=18  bin_pt=16  preci_type=Single  exp_width=8  frac_width=24  optimize=Area  use_rpm=on  dbl_ovrd=off  block_type=sprom
  real1 : xbsIndex_r4/ROM  depth=8  initVector=real(exp(-j*2*pi*(8:15)/16))  distributed_mem=Block RAM  rst=off  init_reg=0  en=off  latency=2  gui_display_data_type=Fixed-point  arith_type="Signed  (2's comp)"  n_bits=18  bin_pt=16  preci_type=Single  exp_width=8  frac_width=24  optimize=Area  use_rpm=on  dbl_ovrd=off  block_type=sprom
  real3 : xbsIndex_r4/ROM  depth=8  initVector=real(exp(-j*2*pi*(0:7)/16))  distributed_mem=Block RAM  rst=off  init_reg=0  en=off  latency=2  gui_display_data_type=Fixed-point  arith_type="Signed  (2's comp)"  n_bits=18  bin_pt=16  preci_type=Single  exp_width=8  frac_width=24  optimize=Area  use_rpm=on  dbl_ovrd=off  block_type=sprom
  slice1 : xbsIndex_r4/BitBasher  bitexpr="out ={17'b0,  indx, im, re }"  display_expr=off  sr_1=out  arith_type1=Unsigned  bin_pt1=0  sr_2=2  arith_type2="Signed  (2's comp)"  bin_pt2=16  sr_3=3  arith_type3=Unsigned  bin_pt3=0  sr_4=4  arith_type4=Unsigned  bin_pt4=0  dbl_ovrd=off  block_type=bitbasher
  slice5 : xbsIndex_r4/BitBasher  bitexpr=out ={19'b0, tlast, indx, im[20:0], re[20:0] }  display_expr=off  sr_1=out  arith_type1=Unsigned  bin_pt1=0  sr_2=2  arith_type2="Signed  (2's comp)"  bin_pt2=16  sr_3=3  arith_type3=Unsigned  bin_pt3=0  sr_4=4  arith_type4=Unsigned  bin_pt4=0  dbl_ovrd=off  block_type=bitbasher
  slice6 : xbsIndex_r4/BitBasher  bitexpr=|  display_expr=off  sr_1=im_out  arith_type1="Signed  (2's comp)"  bin_pt1=17  sr_2=re_out  arith_type2="Signed  (2's comp)"  bin_pt2=17  sr_3=indx  arith_type3=Unsigned  bin_pt3=0  sr_4=tlast  arith_type4=Unsigned  bin_pt4=0  dbl_ovrd=off  block_type=bitbasher
      | im_out ={ in[39:22] }
      | re_out = { in[18:1] }
      | indx    = { in[44:42] } 
      | tlast     = { in[45] }
  slice7 : xbsIndex_r4/BitBasher  bitexpr=out ={19'b0, tlast, indx, im[20:0], re[20:0] }  display_expr=off  sr_1=out  arith_type1=Unsigned  bin_pt1=0  sr_2=2  arith_type2="Signed  (2's comp)"  bin_pt2=16  sr_3=3  arith_type3=Unsigned  bin_pt3=0  sr_4=4  arith_type4=Unsigned  bin_pt4=0  dbl_ovrd=off  block_type=bitbasher
  slice8 : xbsIndex_r4/BitBasher  bitexpr=|  display_expr=off  sr_1=im_out  arith_type1="Signed  (2's comp)"  bin_pt1=17  sr_2=re_out  arith_type2="Signed  (2's comp)"  bin_pt2=17  sr_3=indx  arith_type3=Unsigned  bin_pt3=0  sr_4=tlast  arith_type4=Unsigned  bin_pt4=0  dbl_ovrd=off  block_type=bitbasher
      | im_out ={ in[39:22] }
      | re_out = { in[18:1] }
      | indx    = { in[44:42] } 
      | tlast     = { in[45] }
  valid0 : Outport
  re0 : Outport  Port=2
  im0 : Outport  Port=3
  indx0 : Outport  Port=4
  valid1 : Outport  Port=5
  re1 : Outport  Port=6
  im1 : Outport  Port=7
  indx1 : Outport  Port=8
  wires:
  Register38/1 -> channel_select1/2(data_valid)
  Register37/1 -> FIR Compiler 7.2 2/4
  Register36/1 -> FIR Compiler 7.2 3/4
  Register35/1 -> FIR Compiler 7.2 2/3
  Register34/1 -> FIR Compiler 7.2 3/3
  In2/1 -> BitBasher3/1
  Register31/1 -> Complex Multiplier 6.0 3/1
  Register30/1 -> Complex Multiplier 6.0 3/2
  Register29/1 -> Complex Multiplier 6.0 3/3
  Register28/1 -> Complex Multiplier 6.0 3/4
  imag3/1 -> Complex Multiplier 6.0 3/5
  real3/1 -> Complex Multiplier 6.0 3/6
  Register25/1 -> Complex Multiplier 6.0 2/1
  Register24/1 -> Complex Multiplier 6.0 2/2
  Register16/1 -> Complex Multiplier 6.0 2/3
  Register5/1 -> Complex Multiplier 6.0 2/4
  imag1/1 -> Complex Multiplier 6.0 2/5
  real1/1 -> Complex Multiplier 6.0 2/6
  FIR Compiler 7.2 2/6 -> slice5/1, Gateway Out1/1
  slice6/1 -> Fast Fourier Transform 9.0 2/3
  Gateway Out2/1 -> Scope/2
  Gateway Out1/1 -> Scope/1
  Fast Fourier Transform 9.0 2/5 -> imag3/1, real3/1, imag1/1, real1/1
  FIFO2/1 -> Logical3/2
  FIFO7/3 -> Terminator24/1
  Fast Fourier Transform 9.0 2/13 -> Terminator23/1
  Fast Fourier Transform 9.0 2/12 -> Terminator22/1
  Fast Fourier Transform 9.0 2/11 -> Terminator20/1
  Fast Fourier Transform 9.0 2/10 -> Terminator19/1
  Fast Fourier Transform 9.0 2/9 -> Terminator18/1
  Fast Fourier Transform 9.0 2/8 -> Terminator17/1
  Fast Fourier Transform 9.0 2/7 -> Terminator16/1
  Fast Fourier Transform 9.0 3/13 -> Terminator15/1
  Fast Fourier Transform 9.0 3/12 -> Terminator14/1
  Fast Fourier Transform 9.0 3/11 -> Terminator13/1
  Fast Fourier Transform 9.0 3/10 -> Terminator12/1
  Fast Fourier Transform 9.0 3/9 -> Terminator11/1
  Fast Fourier Transform 9.0 3/8 -> Terminator10/1
  Fast Fourier Transform 9.0 3/7 -> Terminator2/1
  FIFO4/3 -> Terminator1/1
  FIFO2/3 -> Terminator/1
  Split3/3 -> Delay4/1
  FIFO1/3 -> Fast Fourier Transform 9.0 3/7
  FIFO6/3 -> Fast Fourier Transform 9.0 2/7
  FIFO1/2 -> Register23/1
  FIFO1/1 -> Logical2/2
  Split9/3 -> indx0/1
  Split9/2 -> im0/1
  Split9/1 -> re0/1
  Logical2/1 -> valid0/1
  Register23/1 -> Split9/1
  Delay2/1 -> FIFO1/2
  Split4/1 -> FIFO1/3
  AddSub7/1 -> Split4/3
  AddSub6/1 -> Split4/1
  Delay4/1 -> Split4/2, Split5/2
  Logical1/1 -> Delay2/1
  Register18/1 -> AddSub7/2
  Register17/1 -> AddSub6/2
  Split3/2 -> AddSub7/1, AddSub1/1
  Split3/1 -> AddSub6/1, AddSub5/1
  Register22/1 -> Split3/1
  FIFO7/1 -> Logical1/2
  FIFO7/2 -> Register22/1
  slice1/1 -> Register32/1
  Register1/1 -> Register33/1
  Register20/1 -> slice1/3
  Register21/1 -> slice1/2
  Register2/1 -> slice1/1
  Fast Fourier Transform 9.0 3/5 -> Register21/1
  Fast Fourier Transform 9.0 3/6 -> Register21/2, Register20/2, Register2/2, Register1/1
  Fast Fourier Transform 9.0 3/4 -> Register20/1
  Fast Fourier Transform 9.0 3/3 -> Register2/1
  BitBasher2/1 -> Register36/1
  BitBasher3/1 -> Register34/1
  channel_select1/3(t_last) -> FIR Compiler 7.2 2/2, FIR Compiler 7.2 2/6, FIR Compiler 7.2 3/6, FIR Compiler 7.2 3/2
  Convert2/1 -> Fast Fourier Transform 9.0 3/6
  Fast Fourier Transform 9.0 3/1 -> Fast Fourier Transform 9.0 3/2
  FFT3/1 -> Fast Fourier Transform 9.0 3/1
  slice8/4 -> Convert2/1
  Logical3/1 -> Fast Fourier Transform 9.0 3/5
  slice8/2 -> Fast Fourier Transform 9.0 3/4
  slice8/1 -> Fast Fourier Transform 9.0 3/3
  Register19/1 -> slice8/1
  FIFO2/2 -> Register19/1
  Fast Fourier Transform 9.0 3/2 -> Logical3/1, FIFO2/1
  FIR Compiler 7.2 2/11 -> Terminator21/1
  FIR Compiler 7.2 2/10 -> Terminator9/1
  FIR Compiler 7.2 2/9 -> Terminator8/1
  FIR Compiler 7.2 2/8 -> Terminator7/1
  FIR Compiler 7.2 3/11 -> Terminator6/1
  FIR Compiler 7.2 3/10 -> Terminator5/1
  FIR Compiler 7.2 3/9 -> Terminator4/1
  FIR Compiler 7.2 3/8 -> Terminator3/1
  FIR Compiler 7.2 3/3 -> FIFO2/2
  slice7/1 -> FIFO2/3
  FIR Compiler 7.2 3/4 -> slice7/4
  FIR Compiler 7.2 3/5 -> slice7/2
  FIR Compiler 7.2 3/7 -> slice7/3
  FIR Compiler 7.2 3/6 -> slice7/1
  FIR Compiler 7.2 3/2 -> Logical/1
  FIR Compiler 7.2 3/1 -> Logical/2
  FIR Compiler 7.2 2/2 -> Logical/3
  FIR Compiler 7.2 2/1 -> Logical/4
  Complex Multiplier 6.0 3/3 -> Register18/1
  Complex Multiplier 6.0 3/2 -> Register17/1
  Complex Multiplier 6.0 3/1 -> FIFO7/1, Logical1/1
  Register14/1 -> Register30/1
  Register15/1 -> Register29/1
  Split6/3 -> indx1/1
  Split6/2 -> im1/1
  Split6/1 -> re1/1
  Logical7/1 -> valid1/1
  Register13/1 -> Split6/1
  FIFO6/2 -> Register13/1
  FIFO6/1 -> Logical7/2
  Delay1/1 -> FIFO6/2
  Split5/1 -> FIFO6/3
  AddSub1/1 -> Split5/3
  AddSub5/1 -> Split5/1
  Register10/1 -> Delay1/1
  Register11/1 -> AddSub5/2
  Register12/1 -> AddSub1/2
  Complex Multiplier 6.0 2/1 -> Register10/1
  Complex Multiplier 6.0 2/2 -> Register11/1
  Complex Multiplier 6.0 2/3 -> Register12/1
  Register7/1 -> Register5/1, Register25/1, Register31/1, Register28/1
  Register8/1 -> Register24/1
  Register9/1 -> Register16/1
  Fast Fourier Transform 9.0 2/6 -> Register7/1, Register9/2, Register15/2, Register14/2, Register8/2
  Fast Fourier Transform 9.0 2/4 -> Register9/1, Register15/1
  Fast Fourier Transform 9.0 2/3 -> Register8/1, Register14/1
  Convert1/1 -> Fast Fourier Transform 9.0 2/6
  Fast Fourier Transform 9.0 2/1 -> Fast Fourier Transform 9.0 2/2
  FFT2/1 -> Fast Fourier Transform 9.0 2/1
  slice6/4 -> Convert1/1
  FIR Compiler 7.2 2/4 -> slice5/4
  Logical6/1 -> Fast Fourier Transform 9.0 2/5
  slice6/2 -> Fast Fourier Transform 9.0 2/4
  Register6/1 -> slice6/1
  FIFO4/2 -> Register6/1
  Fast Fourier Transform 9.0 2/2 -> FIFO4/1, Logical6/1
  FIFO4/1 -> Logical6/2
  FIR Compiler 7.2 2/3 -> FIFO4/2
  slice5/1 -> FIFO4/3
  FIR Compiler 7.2 2/5 -> slice5/2
  FIR Compiler 7.2 2/7 -> slice5/3, Gateway Out2/1
  Logical/1 -> channel_select1/1(tready)
  In1/1 -> Register38/1
  BitBasher2/2 -> Register37/1
  In3/1 -> BitBasher2/1
  BitBasher3/2 -> Register35/1
  channel_select1/1(tvalid) -> FIR Compiler 7.2 2/1, FIR Compiler 7.2 2/5, FIR Compiler 7.2 3/1, FIR Compiler 7.2 3/5
  channel_select1/2(tdata_fsel) -> FIR Compiler 7.2 3/7, FIR Compiler 7.2 2/7
  t_ready/1 -> FIFO6/1, Logical7/1, FIFO1/1, Logical2/1
  Register32/1 -> FIFO7/3
  Register33/1 -> FIFO7/2
